simulink model "TesteDegrauMinQuadSimulink"  (R2015a)
settings: Solver=ode45  StartTime=0.0  StopTime=30  RelTol=1e-3
values from neighbouring files (symbols this model uses):
  T = 0.04    [Minimos_Quadrados.m]    (also in TesteDegrauMinQuad.m = 0.03)
  tf_analogico = d2c(tf_digital)    [Minimos_Quadrados.m]    (also in TesteDegrauMinQuad.m)
  tf_digital = MinimosQuadrados(N, y, u, T, ordem)    [Minimos_Quadrados.m]    (also in TesteDegrauMinQuad.m)
settings Model: Creator=Lucas  LastModifiedBy=Lucas

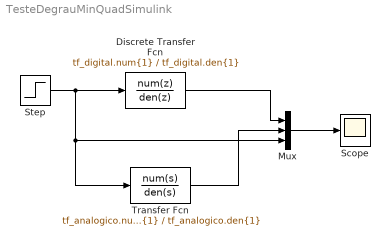
== system TesteDegrauMinQuadSimulink ==
  Discrete Transfer Fcn : DiscreteTransferFcn  Numerator=tf_digital.num{1}  Denominator=tf_digital.den{1}  SampleTime=T
  Mux : Mux  Inputs=3
  Scope : Scope
  Step : Step  Time=11  After=10  SampleTime=T
  Transfer Fcn : TransferFcn  Numerator=tf_analogico.num{1}  Denominator=tf_analogico.den{1}
  wires:
  Discrete Transfer Fcn/1 -> Mux/1
  Step/1 -> Transfer Fcn/1, Mux/3, Discrete Transfer Fcn/1
  Transfer Fcn/1 -> Mux/2
  Mux/1 -> Scope/1
